simulink model "GravityModel"  (R2023b)
settings: Solver=FixedStepAuto  StartTime=0.0  StopTime=10.0  FixedStep=0.001  RelTol=1e-3
model workspace (MAT data in the model file):
  orbit_altitude = Simulink.Parameter
  orbit_altitude.Value = 450000
  orbit_altitude.DataType = 'auto'
  orbit_altitude.Complexity = 'real'
  orbit_altitude.Dimensions = [1 1]
  r_earth = Simulink.Parameter
  r_earth.Value = 6378100
  r_earth.DataType = 'auto'
  r_earth.Complexity = 'real'
  r_earth.Dimensions = [1 1]
  vel_init = 7640
settings Model: Creator=andrea  LastModifiedBy=andrea
settings ModelReferenceCC: UseModelRefSolver=on

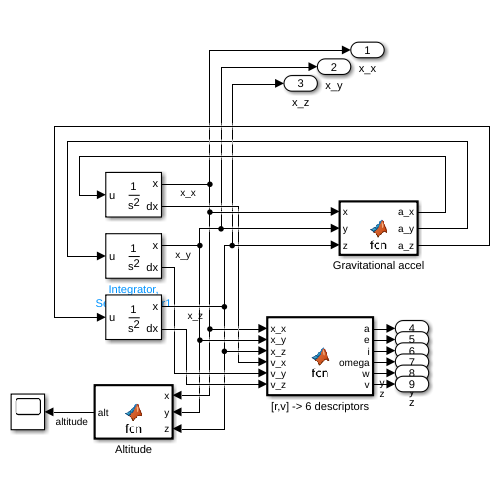
[thumbnail: Simulink's stored preview of the top-level diagram]
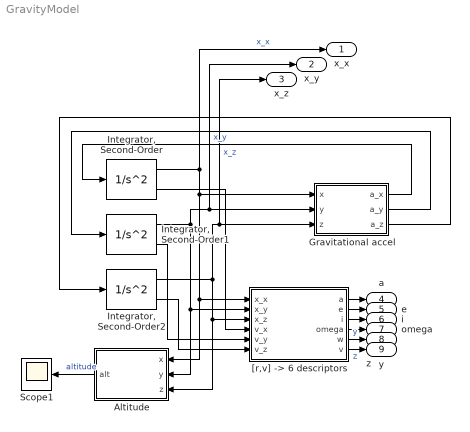
== system GravityModel ==
  Altitude : MATLAB Function  TreatAsAtomicUnit=on
  Gravitational accel : MATLAB Function  TreatAsAtomicUnit=on
  "Integrator, Second-Order" : SecondOrderIntegrator  ICX=0  ICDXDT=5500
  "Integrator, Second-Order1" : SecondOrderIntegrator  ICX=r_earth + orbit_altitude  ICDXDT=0
  "Integrator, Second-Order2" : SecondOrderIntegrator  ICDXDT=5300
  Scope1 : Scope
  "[r,v] -> 6 descriptors" : MATLAB Function  TreatAsAtomicUnit=on
  x_x : Outport
  x_y : Outport  Port=2
  x_z : Outport  Port=3
  a : Outport  Port=4
  e : Outport  Port=5
  i : Outport  Port=6
  omega : Outport  Port=7
  y : Outport  Port=8
  z : Outport  Port=9
  wires:
  "[r,v] -> 6 descriptors"/2(e) -> e/1
  Altitude/1(alt) -> Scope1/1  "altitude"
  "[r,v] -> 6 descriptors"/1(a) -> a/1
  "Integrator, Second-Order1"/2 -> "[r,v] -> 6 descriptors"/5(v_y)
  "[r,v] -> 6 descriptors"/6(v) -> z/1  "z"
  Gravitational accel/3(a_z) -> "Integrator, Second-Order2"/1
  "Integrator, Second-Order1"/1 -> "[r,v] -> 6 descriptors"/2(x_y), Altitude/2(y), x_y/1, Gravitational accel/2(y)  "x_y"
  Gravitational accel/2(a_y) -> "Integrator, Second-Order1"/1
  "[r,v] -> 6 descriptors"/3(i) -> i/1
  Gravitational accel/1(a_x) -> "Integrator, Second-Order"/1
  "Integrator, Second-Order2"/1 -> "[r,v] -> 6 descriptors"/3(x_z), Altitude/3(z), x_z/1, Gravitational accel/3(z)  "x_z"
  "Integrator, Second-Order"/1 -> x_x/1, "[r,v] -> 6 descriptors"/1(x_x), Altitude/1(x), Gravitational accel/1(x)  "x_x"
  "[r,v] -> 6 descriptors"/4(omega) -> omega/1
  "Integrator, Second-Order"/2 -> "[r,v] -> 6 descriptors"/4(v_x)
  "[r,v] -> 6 descriptors"/5(w) -> y/1  "y"
  "Integrator, Second-Order2"/2 -> "[r,v] -> 6 descriptors"/6(v_z)

== matlab function GravityModel/Gravitational accel ==
  data: x input; a_x output; y input; z input; a_y output; a_z output
function [a_x, a_y, a_z] = fcn(x, y, z)
% determine acceleration
d = sqrt(x^2 + y^2 + z^2);
a = -((6.67408*10^-11) * (5.97219*10^24)) / d^2;
% x,y,z unit vector for direction
x1 = x / d;
y1 = y / d;
z1 = z / d;
% x,y,z acceleration vectors
a_x = a * x1;
a_y = a * y1;
a_z = a * z1;

== matlab function GravityModel/[r,v] -> 6 descriptors ==
  data: x_x input; a output; x_y input; x_z input; v_x input; v_y input; v_z input; e output; i output; omega output; w output; v output
function [a, e, i, omega, w, v] = fcn(x_x, x_y, x_z, v_x, v_y, v_z)

% by math magic, we know (SEE RESEARCH FILES\Orbital mechanics.pdf):
% e is the eccentricity vector, that points from apoapsis to periapsis with
% magnitude = orbit's scalar eccentricity; mu is standard gravitational
% parameter: mu = G(m1 + m2), in this case satellite mass is negligible. 

r = [x_x, x_y, x_z];
r_hat = r / norm(r);
r_dot = [v_x, v_y, v_z];
h = cross(r,r_dot);
mu = 3.986004418*10^14;
ecc_vec = (1 / mu) * (cross(r_dot,h) - mu * r_hat);
e = norm(ecc_vec); % e

i = acos(h(3) / norm(h)); % i

spec_mech_e = ((norm(r_dot))^2 / 2) - mu / norm(r);
a = (-mu) / (2 * spec_mech_e); % a

if(i ~= 0)
    n = cross([0,0,1],h);
    omega = acos(n(1) / norm(n)); % omega
    if(n(2) < 0)
        omega = 2*pi - omega;
    end
    
    w = acos(dot(n,ecc_vec) / (norm(n) * e)); % w
    if(ecc_vec(3) < 0)
        w = 2*pi - w;
    end
    
    v = acos(dot(ecc_vec,r) / (norm(r) * e)); % v
    if(dot(r,r_dot) < 0)
        w = 2*pi - w;
    end
else
    omega = 0;
    w = 0;
    v = 0;
end

== matlab function GravityModel/Altitude ==
  data: x input; alt output; y input; z input
function alt = fcn(x, y, z)

alt = sqrt(x^2 + y^2 + z^2) - (6.3781*10^6);
